simulink model "Ass3Q2_2"  (R2018b)
settings: Solver=VariableStepAuto  StartTime=0.0  StopTime=40.0  RelTol=1e-3
values from neighbouring files (symbols this model uses):
  A = [-50,0;0,-50;]    [Adaptive3.m]
  B = [1,0,0;0,1,0]    [Adaptive3.m]
  C = [X(2),X(1)]    [Adaptive3.m]
  D = [X(3),0,1]    [Adaptive3.m]
  flag = 0    [Adaptive3.m]
undefined symbols (not defined in the file or in its folder): ss_mo, ss_pl
settings Model: Creator=bigfoot  LastModifiedBy=bigfoot

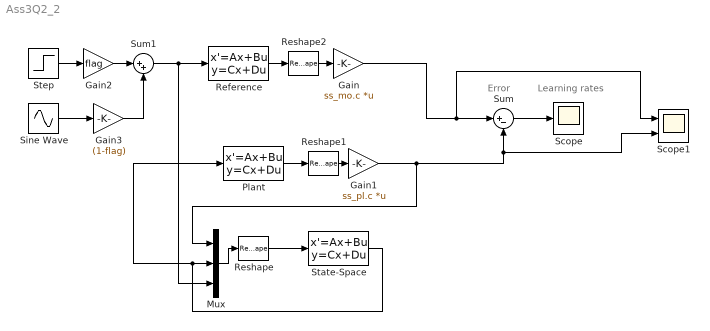
== system Ass3Q2_2 ==
  note: Learning rates
  note: Error
  Gain : Gain  Gain=ss_mo.c  Multiplication=Matrix(K*u)
  Gain1 : Gain  Gain=ss_pl.c  Multiplication=Matrix(K*u)
  Gain2 : Gain  Gain=flag
  Gain3 : Gain  Gain=(1-flag)
  Mux : Mux  Inputs=3
  Plant : StateSpace  A=ss_pl.a  B=ss_pl.b  C=eye(2)  D=[0;0]  InitialCondition=[0,0]
  Reference : StateSpace  A=ss_mo.a  B=ss_mo.b  C=eye(2)  D=[0;0]  InitialCondition=0
  Reshape : Reshape  OutputDimensionality=Column vector (2-D)
  Reshape1 : Reshape  OutputDimensionality=Column vector (2-D)
  Reshape2 : Reshape  OutputDimensionality=Column vector (2-D)
  Scope : Scope
  Scope1 : Scope  NumInputPorts=2
  Sine Wave : Sin  SampleTime=0
  State-Space : StateSpace  A=A  B=B  C=C  D=D  InitialCondition=0
  Step : Step  SampleTime=0
  Sum : Sum  Inputs=|+-
  Sum1 : Sum  Inputs=|++
  wires:
  Gain1/1 -> Mux/1, Scope1/2, Sum/2
  Gain/1 -> Scope1/1, Sum/1
  Sum/1 -> Scope/1
  Mux/1 -> Reshape/1
  Reshape/1 -> State-Space/1
  State-Space/1 -> Plant/1, Mux/2
  Sum1/1 -> Reference/1, Mux/3
  Reference/1 -> Reshape2/1
  Reshape2/1 -> Gain/1
  Plant/1 -> Reshape1/1
  Reshape1/1 -> Gain1/1
  Step/1 -> Gain2/1
  Gain2/1 -> Sum1/1
  Sine Wave/1 -> Gain3/1
  Gain3/1 -> Sum1/2
